simulink model "Continuous_Model_6States"  (R2021b)
settings: Solver=VariableStepAuto  StartTime=0.0  StopTime=1900  RelTol=1e-3
values from neighbouring files (symbols this model uses):
  mu0 = 0    [Continuous_Model_Parameters.m]
  n0 = 0    [Continuous_Model_Parameters.m]
  r0 = 0    [Continuous_Model_Parameters.m]
  s0 = 5    [Continuous_Model_Parameters.m]
  vx0 = 5    [Continuous_Model_Parameters.m]
  vy0 = 0    [Continuous_Model_Parameters.m]
settings Model: Creator=21738394  LastModifiedBy=21738394

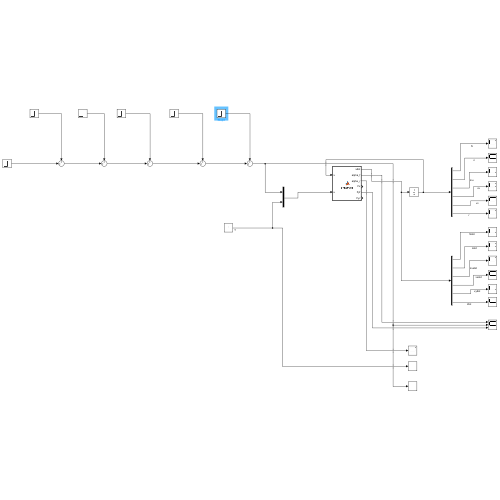
[thumbnail: Simulink's stored preview of the top-level diagram]
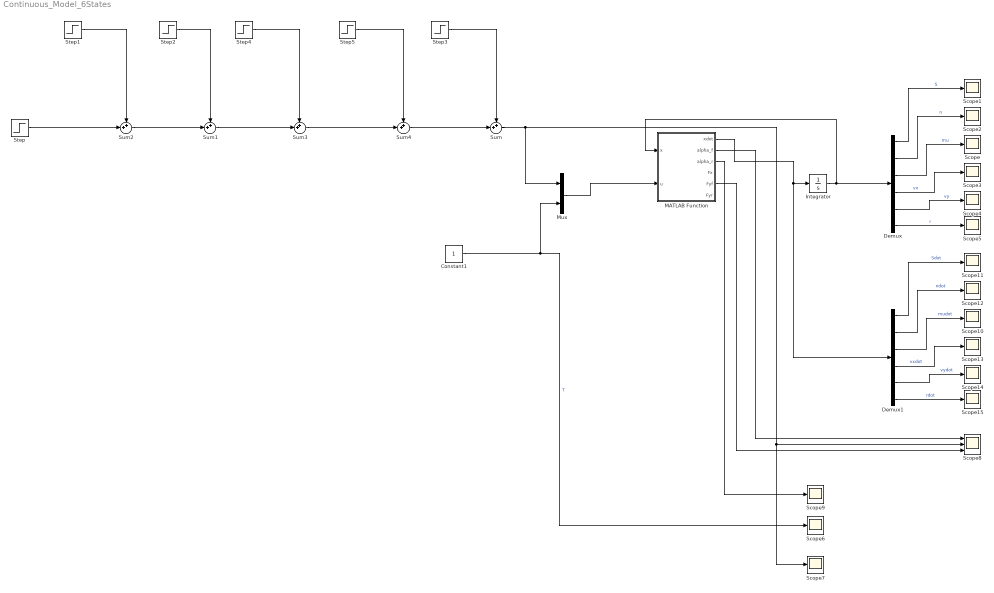
== system Continuous_Model_6States ==
  Constant1 : Constant  SampleTime=-1
  Demux : Demux  Outputs=6
  Demux1 : Demux  Outputs=6
  Integrator : Integrator  InitialCondition=[s0 n0 mu0 vx0 vy0 r0]
  MATLAB Function : MATLAB Function  TreatAsAtomicUnit=on
  Mux : Mux  Inputs=2
  Scope{,1..7,9..15} (15 alike) : Scope
  Scope8 : Scope  NumInputPorts=3
  Step : Step  Time=200  After=0.1  SampleTime=0
  Step1 : Step  Time=400  After=0  SampleTime=0
  Step2 : Step  Time=600  After=0  SampleTime=0
  Step3 : Step  Time=1200  After=0  SampleTime=0
  Step4 : Step  Time=800  After=0  SampleTime=0
  Step5 : Step  Time=1000  After=0  SampleTime=0
  Sum{,1..4} (5 alike) : Sum  Inputs=++|
  wires:
  MATLAB Function/1(xdot) -> Demux1/1, Integrator/1
  Demux/6 -> Scope5/1  "r"
  Constant1/1 -> Mux/2, Scope6/1  "T"
  Integrator/1 -> Demux/1, MATLAB Function/1(x)
  Demux/5 -> Scope4/1  "vy"
  Mux/1 -> MATLAB Function/2(u)
  Demux/4 -> Scope3/1  "vx"
  Demux/2 -> Scope2/1  "n"
  Demux/3 -> Scope/1  "mu"
  Demux/1 -> Scope1/1  "S"
  Sum/1 -> Scope8/2, Scope7/1, Mux/1
  MATLAB Function/2(alpha_f) -> Scope8/1
  MATLAB Function/3(alpha_r) -> Scope9/1
  MATLAB Function/5(Fyf) -> Scope8/3
  Demux1/1 -> Scope11/1  "Sdot"
  Demux1/4 -> Scope13/1  "vxdot"
  Demux1/3 -> Scope10/1  "mudot"
  Demux1/6 -> Scope15/1  "rdot"
  Demux1/5 -> Scope14/1  "vydot"
  Demux1/2 -> Scope12/1  "ndot"
  Step/1 -> Sum2/2
  Step1/1 -> Sum2/1
  Step2/1 -> Sum1/1
  Step3/1 -> Sum/1
  Sum2/1 -> Sum1/2
  Step4/1 -> Sum3/1
  Step5/1 -> Sum4/1
  Sum1/1 -> Sum3/2
  Sum3/1 -> Sum4/2
  Sum4/1 -> Sum/2

== matlab function Continuous_Model_6States/MATLAB Function ==
  data: x input; u input; xdot output; alpha_f output; alpha_r output; Fx output; Fyf output; Fyr output
function [xdot, alpha_f, alpha_r, Fx, Fyf, Fyr]= dynamics(x,u)

s    = x(1);
n    = x(2);
mu   = x(3);
vx   = x(4);
vy   = x(5);
r    = x(6);

str   = u(1);
T     = u(2);

Ks = 0.5;

Bf = 10;
Br = 10;
Cf = 1.9;
Cr = 1.9;
Dr = 1;
Df = 1;
Cm = 5;
Cr0 = 0.0;
Cr2 = 0.2;
l_f = 0.15875;
l_r = 0.17145;
mass = 3.74;
Iz = 0.04712;
FN_r = (mass*9.81*l_r)/(l_r+l_f);
FN_f =(mass*9.81*l_f)/(l_r+l_f);
p_tv = 0;


Fx = (Cm*T) - Cr0 - (Cr2*(vx^2));
alpha_f = -atan((vy + l_f*r)/vx) + str;
Fyf = FN_f*Df*sin(Cf*atan(Bf*alpha_f));
alpha_r = -atan((vy - l_r*r)/vx) ;
Fyr = FN_r*Dr*sin(Cr*atan(Br*alpha_r));
Mtv = p_tv*(((tan(str)*vx)/(l_r + l_f)) - r);

sdot = ((vx*cos(mu)) - (vy*sin(mu)))/(1 - n*Ks);
ndot = (vx*sin(mu)) + (vy*cos(mu));
mudot = r - (Ks*sdot);
vxdot = (1/mass)*(Fx - Fyf*sin(str) + mass*vy*r);
vydot = (1/mass)*(Fyr + Fyr*cos(str) - mass*vx*r);
rdot = (1/Iz) * (Fyf*l_f*cos(str) - Fyr*l_r + Mtv)';

xdot = [sdot ndot mudot vxdot vydot rdot];
